simulink model "LawnMowerPlant"  (R2026a)
settings: Solver=ode45  StopTime=simStopTime
settings Model: Creator=akifd  LastModifiedBy=akifd

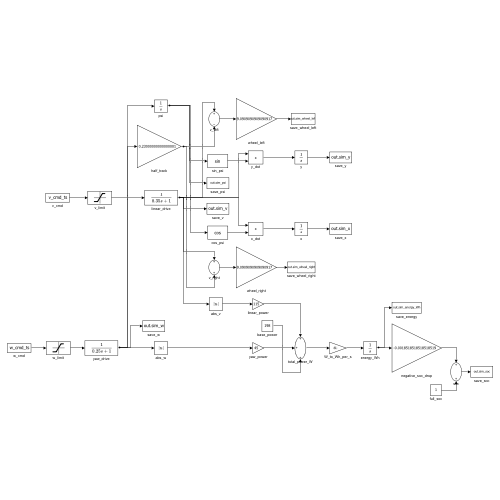
[thumbnail: Simulink's stored preview of the top-level diagram]
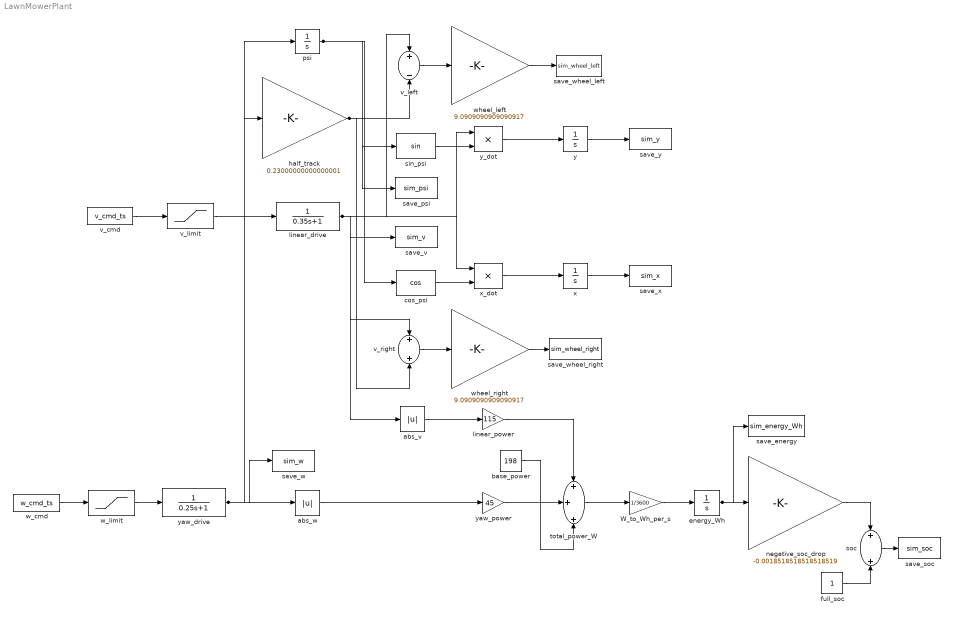
== system LawnMowerPlant ==
  W_to_Wh_per_s : Gain  Gain=1/3600
  abs_v : Abs  SaturateOnIntegerOverflow=off
  abs_w : Abs  SaturateOnIntegerOverflow=off
  base_power : Constant  Value=198
  cos_psi : Trigonometry  Operator=cos
  energy_Wh : Integrator
  full_soc : Constant
  half_track : Gain  Gain=0.23000000000000001
  linear_drive : TransferFcn  Numerator=1  Denominator=[0.35 1]
  linear_power : Gain  Gain=115
  negative_soc_drop : Gain  Gain=-0.0018518518518518519
  psi : Integrator
  save_energy : ToWorkspace  VariableName=sim_energy_Wh  SaveFormat=Timeseries  SampleTime=-1
  save_psi : ToWorkspace  VariableName=sim_psi  SaveFormat=Timeseries  SampleTime=-1
  save_soc : ToWorkspace  VariableName=sim_soc  SaveFormat=Timeseries  SampleTime=-1
  save_v : ToWorkspace  VariableName=sim_v  SaveFormat=Timeseries  SampleTime=-1
  save_w : ToWorkspace  VariableName=sim_w  SaveFormat=Timeseries  SampleTime=-1
  save_wheel_left : ToWorkspace  VariableName=sim_wheel_left  SaveFormat=Timeseries  SampleTime=-1
  save_wheel_right : ToWorkspace  VariableName=sim_wheel_right  SaveFormat=Timeseries  SampleTime=-1
  save_x : ToWorkspace  VariableName=sim_x  SaveFormat=Timeseries  SampleTime=-1
  save_y : ToWorkspace  VariableName=sim_y  SaveFormat=Timeseries  SampleTime=-1
  sin_psi : Trigonometry
  soc : Sum
  total_power_W : Sum  Inputs=+++
  v_cmd : FromWorkspace  VariableName=v_cmd_ts
  v_left : Sum  Inputs=+-
  v_limit : Saturate  UpperLimit=0.80000000000000004  LowerLimit=-0.80000000000000004
  v_right : Sum
  w_cmd : FromWorkspace  VariableName=w_cmd_ts
  w_limit : Saturate  UpperLimit=0.90000000000000002  LowerLimit=-0.90000000000000002
  wheel_left : Gain  Gain=9.0909090909090917
  wheel_right : Gain  Gain=9.0909090909090917
  x : Integrator  InitialCondition=0.20000000000000001
  x_dot : Product  Inputs=**
  y : Integrator  InitialCondition=0.20000000000000001
  y_dot : Product  Inputs=**
  yaw_drive : TransferFcn  Numerator=1  Denominator=[0.25 1]
  yaw_power : Gain  Gain=45
  wires:
  yaw_drive/1 -> psi/1, abs_w/1, half_track/1, save_w/1
  x/1 -> save_x/1
  yaw_power/1 -> total_power_W/2
  w_cmd/1 -> w_limit/1
  w_limit/1 -> yaw_drive/1
  half_track/1 -> v_right/2, v_left/2
  v_cmd/1 -> v_limit/1
  psi/1 -> cos_psi/1, sin_psi/1, save_psi/1
  y/1 -> save_y/1
  v_limit/1 -> linear_drive/1
  linear_drive/1 -> x_dot/1, v_right/1, y_dot/1, save_v/1, abs_v/1, v_left/1
  abs_w/1 -> yaw_power/1
  v_left/1 -> wheel_left/1
  sin_psi/1 -> y_dot/2
  cos_psi/1 -> x_dot/2
  v_right/1 -> wheel_right/1
  abs_v/1 -> linear_power/1
  wheel_left/1 -> save_wheel_left/1
  linear_power/1 -> total_power_W/1
  y_dot/1 -> y/1
  x_dot/1 -> x/1
  wheel_right/1 -> save_wheel_right/1
  base_power/1 -> total_power_W/3
  total_power_W/1 -> W_to_Wh_per_s/1
  W_to_Wh_per_s/1 -> energy_Wh/1
  energy_Wh/1 -> negative_soc_drop/1, save_energy/1
  negative_soc_drop/1 -> soc/1
  full_soc/1 -> soc/2
  soc/1 -> save_soc/1
